simulink model "problem3"  (R2013a)
settings: Solver=ode14x  StartTime=0.0  StopTime=10.0  FixedStep=0.0001  RelTol=1e-3
libraries: fl_lib x5, nesl_utility x3, elec_lib x1
settings Model: Creator=Samanth  LastModifiedBy=Samanth

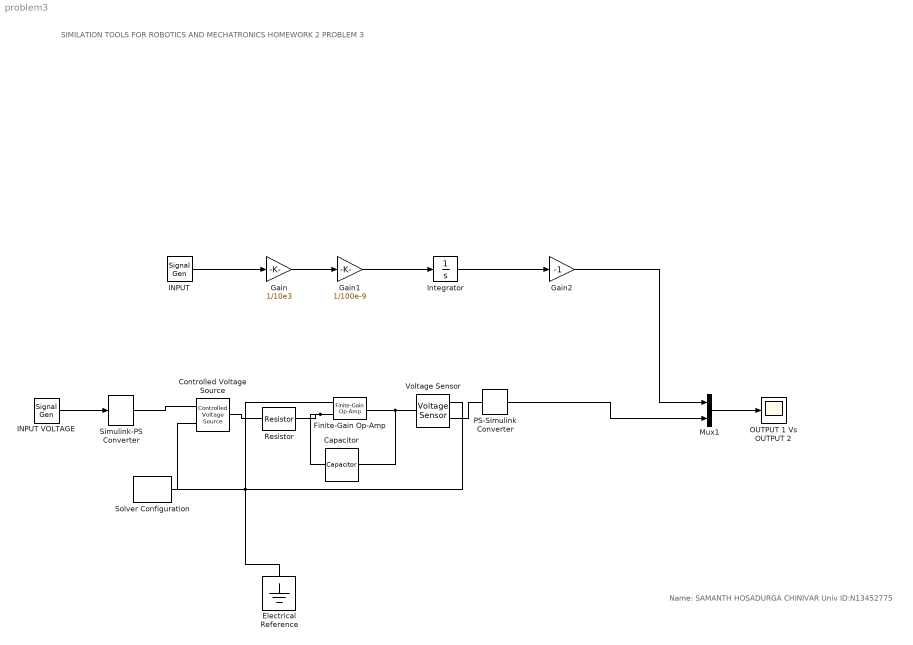
== system problem3 ==
  note: Name: SAMANTH HOSADURGA CHINIVAR
      | Univ ID:N13452775
  note: SIMILATION TOOLS FOR ROBOTICS AND MECHATRONICS
      |                                                                                                                                HOMEWORK 2
      |                                                                                                                              PROBLEM 3
  Capacitor : fl_lib/Electrical/Electrical Elements/Capacitor  c=100 nF  v0=0 V  r=1e-6 Ohm  g=0 1/Ohm  i_Log=off  v_Log=off  vc_Log=off  LocalVarNames=|i|v|vc  LocalVarDescs=|i|v|Internal variable for voltage across capacitor term  LocalVarLogging=[0 0 0]
  Controlled Voltage Source : fl_lib/Electrical/Electrical Sources/Controlled Voltage Source  i_Log=off  v_Log=off  LocalVarNames=|i|v  LocalVarDescs=|i|v  LocalVarLogging=[0 0]
  Electrical Reference : fl_lib/Electrical/Electrical Elements/Electrical Reference  i_Log=off  LocalVarNames=|i  LocalVarDescs=|i  LocalVarLogging=0
  Finite-Gain Op-Amp : elec_lib/Integrated Circuits/Finite-Gain Op-Amp  A=200000  Rin=1e+6 Ohm  Rout=100 Ohm  Vmin=-15 V  Vmax=15 V  LocalVarLogging=[]
  Gain : Gain  Gain=1/10e3
  Gain1 : Gain  Gain=1/100e-9
  Gain2 : Gain  Gain=-1
  INPUT : SignalGenerator  WaveForm=square  Frequency=40
  INPUT VOLTAGE : SignalGenerator  WaveForm=square  Frequency=40
  Integrator : Integrator
  Mux1 : Mux  Inputs=2
  OUTPUT 1 Vs OUTPUT 2 : Scope
      settings: YMin=-1  YMax=13  SaveName=ScopeData2
  PS-Simulink Converter : nesl_utility/PS-Simulink Converter  PhysicalDomain=network_engine_domain  SubClassName=ps_output  LeftPortType=input  RightPortType=output  PseudoPeriodic=off  Frequencies=[]  Unit=1  AffineConversion=off
  Resistor : fl_lib/Electrical/Electrical Elements/Resistor  R=10 kOhm  i_Log=off  v_Log=off  LocalVarNames=|i|v  LocalVarDescs=|i|v  LocalVarLogging=[0 0]
  Simulink-PS Converter : nesl_utility/Simulink-PS Converter  PhysicalDomain=network_engine_domain  SubClassName=ps_input  LeftPortType=input  RightPortType=output  PseudoPeriodic=off  Frequencies=[]  NoiseDistribution=none  NoiseParameters=[]  Unit=1  AffineConversion=off  InputFiltering=off  SimscapeFilterOrder=1  InputFilterTimeConstant=0.001  UdotUserProvided=1
  Solver Configuration : nesl_utility/Solver Configuration  PhysicalDomain=network_engine_domain  SubClassName=solver  LeftPortType=input  RightPortType=generic  Accelerate=off  Tones=[]  Harmonics=[]  SimulateNoise=off  Profile=off  UseLocalSampling=off  EnableSwitchedLinearOptims=on  FrequencyDomain=off  UseCCode=off  UseNewInitialization=off  DoDC=off  ResidualTolerance=1e-09  UseLocalSolver=off  LocalSolverChoice=NE_BACKWARD_EULER_ADVANCER  LocalSolverSampleTime=0.001  DoFixedCost=off  MaxNonlinIter=3  MaxModeIter=2  LinearAlgebra=Sparse  DelaysMemoryBudget=1024
  Voltage Sensor : fl_lib/Electrical/Electrical Sensors/Voltage Sensor  i1_Log=off  v1_Log=off  LocalVarNames=|i1|v1  LocalVarDescs=|i1|v1  LocalVarLogging=[0 0]
  wires:
  Gain/1 -> Gain1/1
  Gain1/1 -> Integrator/1
  Integrator/1 -> Gain2/1
  INPUT/1 -> Gain/1
  INPUT VOLTAGE/1 -> Simulink-PS Converter/1
  PS-Simulink Converter/1 -> Mux1/2
  Gain2/1 -> Mux1/1
  Mux1/1 -> OUTPUT 1 Vs OUTPUT 2/1
  connections:
  Finite-Gain Op-Amp/LConn2 -- Resistor/RConn1 -- Capacitor/LConn1
  Electrical Reference/LConn1 -- Controlled Voltage Source/RConn2 -- Solver Configuration/RConn1 -- Voltage Sensor/RConn2 -- Finite-Gain Op-Amp/LConn1
  Voltage Sensor/LConn1 -- Capacitor/RConn1 -- Finite-Gain Op-Amp/RConn1
  Voltage Sensor/RConn1 -- PS-Simulink Converter/LConn1
  Resistor/LConn1 -- Controlled Voltage Source/LConn1
  Simulink-PS Converter/RConn1 -- Controlled Voltage Source/RConn1
